simulink model "mod3_1plus1plus1MASH"  (Simulink 8.1)
settings: Solver=FixedStepDiscrete  StartTime=0.0  StopTime=1  RelTol=1e-3
undefined symbols (not defined in the file): dfilt, Fs, modctrl
libraries: dspsigops x5, dsparch4 x2, dspsrcs4 x2
settings Model: Creator=amyles  LastModifiedBy=amyles
settings DataIOCC: LimitDataPoints=off  MaxDataPoints=50000  SignalLoggingSaveFormat=Dataset
settings OptimizationCC: InlineParams=on
settings DebuggingCC: StrictBusMsg=Warning
settings ModelReferenceCC: ModelReferenceNumInstancesAllowed=Single

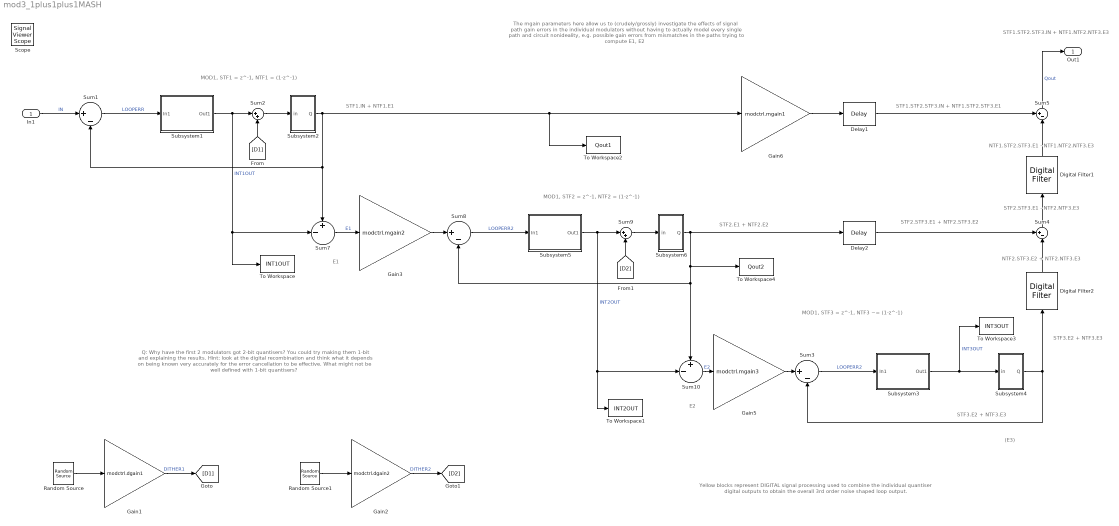
== system mod3_1plus1plus1MASH ==
  note: MOD1, STF1 = z^-1, NTF1 = (1-z^-1)
  note: E1
  note: E2
  note: STF1.IN + NTF1.E1
  note: STF2.E1 + NTF2.E2
  note: STF3.E2 + NTF3.E3
  note: NTF2.STF3.E2 + NTF2.NTF3.E3
  note: STF2.STF3.E1 + NTF2.STF3.E2
  note: STF2.STF3.E1 - NTF2.NTF3.E3
  note: NTF1.STF2.STF3.E1 - NTF1.NTF2.NTF3.E3
  note: STF1.STF2.STF3.IN + NTF1.STF2.STF3.E1
  note: MOD1, STF2 = z^-1, NTF2 = (1-z^-1)
  note: MOD1, STF3 = z^-1, NTF3 ~= (1-z^-1)
  note: STF1.STF2.STF3.IN + NTF1.NTF2.NTF3.E3
  note: Q: Why have the first 2 modulators got 2-bit quantisers?
      |
      | You could try making them 1-bit and explaining the results.
      | Hint: look at the digital recombination and think what it
      | depends on being known very accurately for the error
      | cancellation to be effective.
      | What might not be well defined with 1-bit quantisers?
  note: The mgain parameters here allow us to (crudely/grossly) investigate the effects of signal path gain
      | errors in the individual modulators without having to actually model every single path and
      | circuit nonideality, e.g. possible gain errors from mismatches in the paths trying to compute E1, E2
  note: (E3)
  note: Yellow blocks represent DIGITAL signal processing used to combine the individual
      | quantiser digital outputs to obtain the overall 3rd order noise shaped loop output.
  note: STF3.E2 + NTF3.E3
  In1 : Inport
  Delay1 : dspsigops/Delay  InputProcessing=Columns as channels (frame based)  dly_unit=Samples  delay=2  ic_detail=off  dif_ic_for_ch=off  dif_ic_for_dly=off  ic=0  reset_popup=None
      settings: AttributesFormatString=STF2.STF3
  Delay2 : dspsigops/Delay  InputProcessing=Columns as channels (frame based)  dly_unit=Samples  delay=1  ic_detail=off  dif_ic_for_ch=off  dif_ic_for_dly=off  ic=0  reset_popup=None
      settings: AttributesFormatString=STF3
  Digital Filter1 : dsparch4/Digital Filter  TypePopup=FIR (all zeros)  IIRFiltStruct=Direct form II transposed  AllPoleFiltStruct=Direct form  FIRFiltStruct=Direct form  CoeffSource=Specify via dialog  NumCoeffs=[1 -1]  DenCoeffs=[1 0.1]  BiQuadCoeffs=[1 0.3 0.4 1 0.1 0.2]  LatticeCoeffs=[0.2 0.4]  denIgnore=on  FiltPerSampPopup=One filter per frame  IC=0  ICnum=0  ICden=0  roundingMode=Floor  overflowMode=off  ScaleValues=1  scaleValueFracLength=14  stageInFracLength=15  stageOutFracLength=15  FilterSource=Specify via dialog  dfiltObjectName=dfilt.dffir([1 2 1])  InputProcessing=Columns as channels (frame based)
      settings: AttributesFormatString=NTF1 = (1-z^-1)
  Digital Filter2 : dsparch4/Digital Filter  TypePopup=FIR (all zeros)  IIRFiltStruct=Direct form II transposed  AllPoleFiltStruct=Direct form  FIRFiltStruct=Direct form  CoeffSource=Specify via dialog  NumCoeffs=[1 -1]  DenCoeffs=[1 0.1]  BiQuadCoeffs=[1 0.3 0.4 1 0.1 0.2]  LatticeCoeffs=[0.2 0.4]  denIgnore=on  FiltPerSampPopup=One filter per frame  IC=0  ICnum=0  ICden=0  roundingMode=Floor  overflowMode=off  ScaleValues=1  scaleValueFracLength=14  stageInFracLength=15  stageOutFracLength=15  FilterSource=Specify via dialog  dfiltObjectName=dfilt.dffir([1 2 1])  InputProcessing=Columns as channels (frame based)
      settings: AttributesFormatString=NTF2 = (1-z^-1)
  Gain1 : Gain  Gain=modctrl.dgain1
      settings: AttributesFormatString=Dither level adjust
  Gain2 : Gain  Gain=modctrl.dgain2
      settings: AttributesFormatString=Dither level adjust
  Gain3 : Gain  Gain=modctrl.mgain2
  Gain5 : Gain  Gain=modctrl.mgain3
  Gain6 : Gain  Gain=modctrl.mgain1
  Random Source : dspsrcs4/Random Source  SrcType=Uniform  NormMethod=Ziggurat  CltLength=12  MinVal=-1  MaxVal=1  MeanVal=0  VarVal=1  RepMode=Not repeatable  rawSeed=1  IsInherit=off  SampMode=Discrete  SampTime=1/Fs  SampFrame=1  DataType=Double  OutComplex=Real
      settings: AttributesFormatString=Dither source
  Random Source1 : dspsrcs4/Random Source  SrcType=Uniform  NormMethod=Ziggurat  CltLength=12  MinVal=-1  MaxVal=1  MeanVal=0  VarVal=1  RepMode=Not repeatable  rawSeed=1  IsInherit=off  SampMode=Discrete  SampTime=1/Fs  SampFrame=1  DataType=Double  OutComplex=Real
      settings: AttributesFormatString=Dither source
  Subsystem1 : Subsystem
      settings: AttributesFormatString=Leaky delaying int
  Subsystem2 : Subsystem
      settings: AttributesFormatString=2-bit quantiser
  Subsystem3 : Subsystem
      settings: AttributesFormatString=Leaky delaying int
  Subsystem4 : Subsystem
      settings: AttributesFormatString=1-bit quantiser
  Subsystem5 : Subsystem
      settings: AttributesFormatString=Leaky delaying int
  Subsystem6 : Subsystem
      settings: AttributesFormatString=2-bit quantiser
  Sum1 : Sum  Inputs=|+-
      settings: AttributesFormatString=Modulator input\nloop servo error (input - fbk)
  Sum{4..5,7,10} (4 alike) : Sum  Inputs=+-|
  Sum2 : Sum  Inputs=|++
  Sum3 : Sum  Inputs=|+-
      settings: AttributesFormatString=Modulator input\nloop servo error (input - fbk)
  Sum8 : Sum  Inputs=|+-
      settings: AttributesFormatString=Modulator input\nloop servo error (input - fbk)
  Sum9 : Sum  Inputs=|++
  To Workspace : ToWorkspace  VariableName=INT1OUT  SampleTime=-1
  To Workspace1 : ToWorkspace  VariableName=INT2OUT  SampleTime=-1
  To Workspace2 : ToWorkspace  VariableName=Qout1  SampleTime=-1
  To Workspace3 : ToWorkspace  VariableName=INT3OUT  SampleTime=-1
  To Workspace4 : ToWorkspace  VariableName=Qout2  SampleTime=-1
  Out1 : Outport
  Scope : SignalViewerScope  IOType=viewer  NumInputPorts=4  ZoomMode=xonly  RefreshTime=0.035000
      settings: YMin=-1.25~-0.75~-1.5~-7.5  YMax=1.25~0.75~1.5~7.5
  wires:
  Random Source1/1 -> Gain2/1
  Sum1/1 -> Subsystem1/1(In1)  "LOOPERR"
  Subsystem1/1(Out1) -> Sum2/1, To Workspace/1, Sum7/2  "INT1OUT"
  Sum2/1 -> Subsystem2/1(in)
  In1/1 -> Sum1/1  "IN"
  Random Source/1 -> Gain1/1
  Sum8/1 -> Subsystem5/1(In1)  "LOOPERR2"
  Subsystem5/1(Out1) -> Sum9/1, To Workspace1/1, Sum10/2  "INT2OUT"
  Sum9/1 -> Subsystem6/1(in)
  Subsystem6/1(Q) -> Sum8/2, Sum10/1, To Workspace4/1, Delay2/1
  Sum3/1 -> Subsystem3/1(In1)  "LOOPERR2"
  Subsystem3/1(Out1) -> Subsystem4/1(in), To Workspace3/1  "INT3OUT"
  Sum10/1 -> Gain5/1  "E2"
  Subsystem4/1(Q) -> Sum3/2, Digital Filter2/1
  Subsystem2/1(Q) -> Sum1/2, Sum7/1, Gain6/1, To Workspace2/1
  Digital Filter2/1 -> Sum4/2
  Delay2/1 -> Sum4/1
  Digital Filter1/1 -> Sum5/2
  Delay1/1 -> Sum5/1
  Gain6/1 -> Delay1/1
  Sum4/1 -> Digital Filter1/1
  Sum5/1 -> Out1/1  "Qout"
  Gain1/1 -> [D1]  "DITHER1"
  Gain2/1 -> [D2]  "DITHER2"
  [D1] -> Sum2/2
  [D2] -> Sum9/2
  Sum7/1 -> Gain3/1  "E1"
  Gain3/1 -> Sum8/1
  Gain5/1 -> Sum3/1

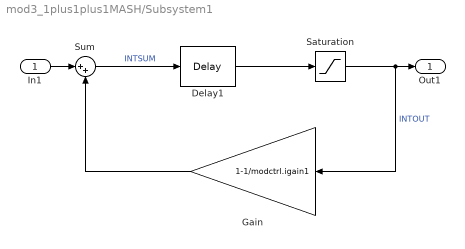
== system mod3_1plus1plus1MASH/Subsystem1 ==
  In1 : Inport
  Delay1 : dspsigops/Delay  InputProcessing=Inherited (this choice will be removed - see release notes)  dly_unit=Samples  delay=1  ic_detail=off  dif_ic_for_ch=off  dif_ic_for_dly=off  ic=0  reset_popup=None
  Gain : Gain  Gain=1-1/modctrl.igain1
      settings: AttributesFormatString=Integrator leakage
  Saturation : Saturate  UpperLimit=modctrl.isat1  LowerLimit=-(modctrl.isat1)
  Sum : Sum  Inputs=|++
      settings: AttributesFormatString=Integrator summer
  Out1 : Outport
  wires:
  Sum/1 -> Delay1/1  "INTSUM"
  Gain/1 -> Sum/2
  Saturation/1 -> Gain/1, Out1/1  "INTOUT"
  Delay1/1 -> Saturation/1
  In1/1 -> Sum/1

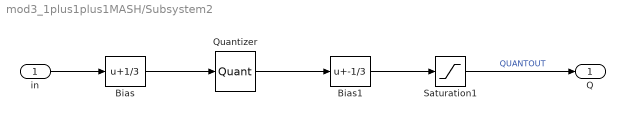
== system mod3_1plus1plus1MASH/Subsystem2 ==
  in : Inport
  Bias : Bias  Bias=1/3
      settings: AttributesFormatString=Need offset to give\nMID-RISE quantiser
  Bias1 : Bias  Bias=-1/3
  Quantizer : Quantizer  QuantizationInterval=2/3  LinearizeAsGain=off
  Saturation1 : Saturate  UpperLimit=1  LowerLimit=-1
      settings: AttributesFormatString=Limit quantiser\noutput to +/-1
  Q : Outport
  wires:
  Saturation1/1 -> Q/1  "QUANTOUT"
  in/1 -> Bias/1
  Bias1/1 -> Saturation1/1
  Quantizer/1 -> Bias1/1
  Bias/1 -> Quantizer/1

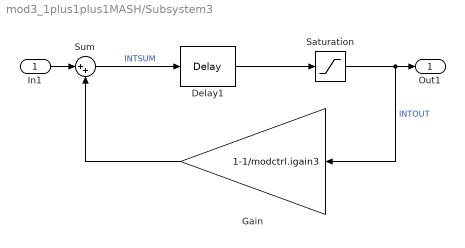
== system mod3_1plus1plus1MASH/Subsystem3 ==
  In1 : Inport
  Delay1 : dspsigops/Delay  InputProcessing=Inherited (this choice will be removed - see release notes)  dly_unit=Samples  delay=1  ic_detail=off  dif_ic_for_ch=off  dif_ic_for_dly=off  ic=0  reset_popup=None
  Gain : Gain  Gain=1-1/modctrl.igain3
      settings: AttributesFormatString=Integrator leakage
  Saturation : Saturate  UpperLimit=modctrl.isat3  LowerLimit=-(modctrl.isat3)
  Sum : Sum  Inputs=|++
      settings: AttributesFormatString=Integrator summer
  Out1 : Outport
  wires:
  Sum/1 -> Delay1/1  "INTSUM"
  Gain/1 -> Sum/2
  Saturation/1 -> Gain/1, Out1/1  "INTOUT"
  Delay1/1 -> Saturation/1
  In1/1 -> Sum/1

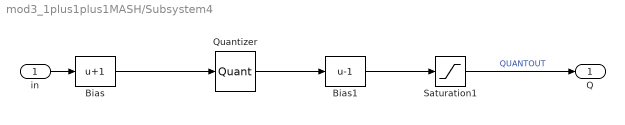
== system mod3_1plus1plus1MASH/Subsystem4 ==
  in : Inport
  Bias : Bias  Bias=1
      settings: AttributesFormatString=Need offset to give\nMID-RISE quantiser
  Bias1 : Bias  Bias=-1
  Quantizer : Quantizer  QuantizationInterval=2  LinearizeAsGain=off
  Saturation1 : Saturate  UpperLimit=1  LowerLimit=-1
      settings: AttributesFormatString=Limit quantiser\noutput to +/-1
  Q : Outport
  wires:
  Saturation1/1 -> Q/1  "QUANTOUT"
  in/1 -> Bias/1
  Bias1/1 -> Saturation1/1
  Quantizer/1 -> Bias1/1
  Bias/1 -> Quantizer/1

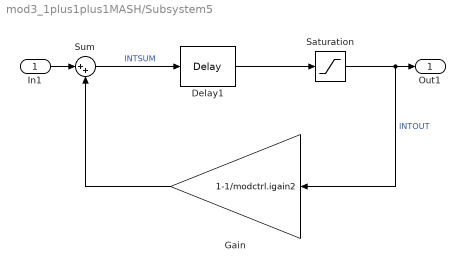
== system mod3_1plus1plus1MASH/Subsystem5 ==
  In1 : Inport
  Delay1 : dspsigops/Delay  InputProcessing=Inherited (this choice will be removed - see release notes)  dly_unit=Samples  delay=1  ic_detail=off  dif_ic_for_ch=off  dif_ic_for_dly=off  ic=0  reset_popup=None
  Gain : Gain  Gain=1-1/modctrl.igain2
      settings: AttributesFormatString=Integrator leakage
  Saturation : Saturate  UpperLimit=modctrl.isat2  LowerLimit=-(modctrl.isat2)
  Sum : Sum  Inputs=|++
      settings: AttributesFormatString=Integrator summer
  Out1 : Outport
  wires:
  In1/1 -> Sum/1
  Delay1/1 -> Saturation/1
  Saturation/1 -> Out1/1, Gain/1  "INTOUT"
  Gain/1 -> Sum/2
  Sum/1 -> Delay1/1  "INTSUM"

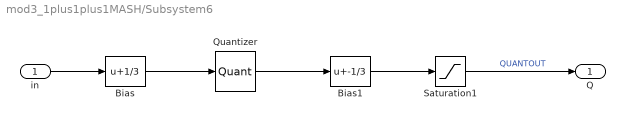
== system mod3_1plus1plus1MASH/Subsystem6 ==
  in : Inport
  Bias : Bias  Bias=1/3
      settings: AttributesFormatString=Need offset to give\nMID-RISE quantiser
  Bias1 : Bias  Bias=-1/3
  Quantizer : Quantizer  QuantizationInterval=2/3  LinearizeAsGain=off
  Saturation1 : Saturate  UpperLimit=1  LowerLimit=-1
      settings: AttributesFormatString=Limit quantiser\noutput to +/-1
  Q : Outport
  wires:
  Bias/1 -> Quantizer/1
  Quantizer/1 -> Bias1/1
  Bias1/1 -> Saturation1/1
  in/1 -> Bias/1
  Saturation1/1 -> Q/1  "QUANTOUT"
